simulink model "v09_twobit_mult"  (R2019b)
settings: Solver=FixedStepAuto  StartTime=0.0  StopTime=inf  FixedStep=1  MaxStep=1  RelTol=1e-3
libraries: simulink x4
settings Model: Creator=MARAT  LastModifiedBy=Marat
settings SFSimCC: CustomCodeUndefinedFunction=UseInterfaceOnly

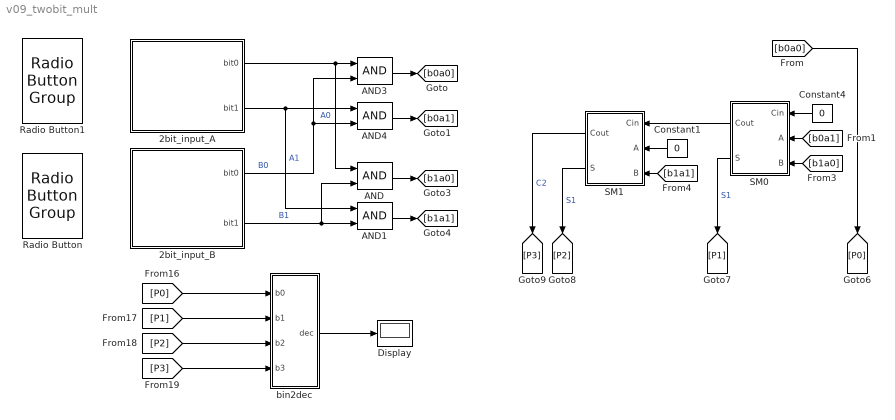
== system v09_twobit_mult ==
  2bit_input_A : Subsystem
      mask Display: image('images\sansA.png'); % Use "Edit Image" on toolstrip to change.
  2bit_input_B : Subsystem
      mask Display: image('images\sansB.png'); % Use "Edit Image" on toolstrip to change.
  AND{,1,3..4} (4 alike) : Logic  AllPortsSameDT=off  OutDataTypeStr=boolean
  Constant1 : Constant  Value=0  OutDataTypeStr=boolean
  Constant4 : Constant  Value=0  OutDataTypeStr=boolean
  Display : Display
  Radio Button : RadioButtonGroup  SelectedLabel=0
      settings: Values={{'0', '1', '2', '3'}, [0 1 2 3]}
  Radio Button1 : RadioButtonGroup  SelectedLabel=0
      settings: Values={{'0', '1', '2', '3'}, [0 1 2 3]}
  SM0 : Subsystem
  SM1 : Subsystem
  bin2dec : Subsystem
  wires:
  Constant4/1 -> SM0/1(Cin)
  [b0a0] -> [P0]
  2bit_input_A/1(bit0) -> AND/1, AND3/1  "A0"
  2bit_input_B/2(bit1) -> AND1/2, AND/2  "B1"
  [P0] -> bin2dec/1(b0)
  [P1] -> bin2dec/2(b1)
  [P2] -> bin2dec/3(b2)
  [P3] -> bin2dec/4(b3)
  bin2dec/1(dec) -> Display/1
  SM0/2(S) -> [P1]  "S1"
  2bit_input_A/2(bit1) -> AND1/1, AND4/1  "A1"
  2bit_input_B/1(bit0) -> AND3/2, AND4/2  "B0"
  AND3/1 -> [b0a0]
  AND4/1 -> [b0a1]
  AND1/1 -> [b1a1]
  AND/1 -> [b1a0]
  [b1a0] -> SM0/3(B)
  [b0a1] -> SM0/2(A)
  [b1a1] -> SM1/3(B)
  Constant1/1 -> SM1/2(A)
  SM0/1(Cout) -> SM1/1(Cin)
  SM1/2(S) -> [P2]  "S1"
  SM1/1(Cout) -> [P3]  "C2"

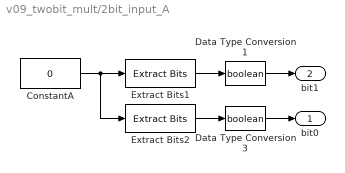
== system v09_twobit_mult/2bit_input_A ==
  ConstantA : Constant  Value=0  OutMin=0  OutMax=3  OutDataTypeStr=uint8
  Data Type Conversion1 : DataTypeConversion  OutDataTypeStr=boolean
  Data Type Conversion3 : DataTypeConversion  OutDataTypeStr=boolean
  Extract Bits1 : simulink/Logic and Bit Operations/Extract Bits  bitsToExtract=Range of bits  numBits=8  bitIdxRange=1  outScalingMode=Treat bit field as an integer
      settings: SourceProductName=Simulink
  Extract Bits2 : simulink/Logic and Bit Operations/Extract Bits  bitsToExtract=Range of bits  numBits=8  bitIdxRange=0  outScalingMode=Treat bit field as an integer
      settings: SourceProductName=Simulink
  bit0 : Outport
  bit1 : Outport  Port=2
  wires:
  ConstantA/1 -> Extract Bits2/1, Extract Bits1/1
  Extract Bits1/1 -> Data Type Conversion1/1
  Extract Bits2/1 -> Data Type Conversion3/1
  Data Type Conversion1/1 -> bit1/1
  Data Type Conversion3/1 -> bit0/1

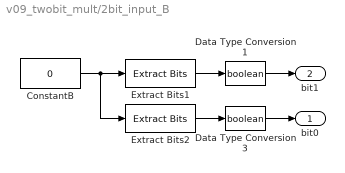
== system v09_twobit_mult/2bit_input_B ==
  ConstantB : Constant  Value=0  OutMin=0  OutMax=3  OutDataTypeStr=uint8
  Data Type Conversion1 : DataTypeConversion  OutDataTypeStr=boolean
  Data Type Conversion3 : DataTypeConversion  OutDataTypeStr=boolean
  Extract Bits1 : simulink/Logic and Bit Operations/Extract Bits  bitsToExtract=Range of bits  numBits=8  bitIdxRange=1  outScalingMode=Treat bit field as an integer
      settings: SourceProductName=Simulink
  Extract Bits2 : simulink/Logic and Bit Operations/Extract Bits  bitsToExtract=Range of bits  numBits=8  bitIdxRange=0  outScalingMode=Treat bit field as an integer
      settings: SourceProductName=Simulink
  bit0 : Outport
  bit1 : Outport  Port=2
  wires:
  Data Type Conversion3/1 -> bit0/1
  Data Type Conversion1/1 -> bit1/1
  Extract Bits2/1 -> Data Type Conversion3/1
  Extract Bits1/1 -> Data Type Conversion1/1
  ConstantB/1 -> Extract Bits1/1, Extract Bits2/1

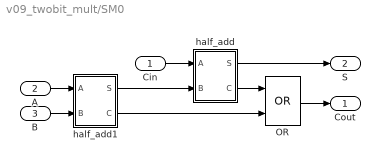
== system v09_twobit_mult/SM0 ==
  Cin : Inport
  A : Inport  Port=2
  B : Inport  Port=3
  OR : Logic  Operator=OR  AllPortsSameDT=off  OutDataTypeStr=boolean
  half_add : Subsystem
  half_add1 : Subsystem
  Cout : Outport
  S : Outport  Port=2
  wires:
  half_add/1(S) -> S/1
  A/1 -> half_add1/1(A)
  half_add/2(C) -> OR/1
  half_add1/1(S) -> half_add/2(B)
  B/1 -> half_add1/2(B)
  Cin/1 -> half_add/1(A)
  OR/1 -> Cout/1
  half_add1/2(C) -> OR/2

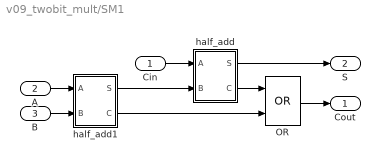
== system v09_twobit_mult/SM1 ==
  Cin : Inport
  A : Inport  Port=2
  B : Inport  Port=3
  OR : Logic  Operator=OR  AllPortsSameDT=off  OutDataTypeStr=boolean
  half_add : Subsystem
  half_add1 : Subsystem
  Cout : Outport
  S : Outport  Port=2
  wires:
  half_add1/2(C) -> OR/2
  OR/1 -> Cout/1
  Cin/1 -> half_add/1(A)
  B/1 -> half_add1/2(B)
  half_add1/1(S) -> half_add/2(B)
  half_add/2(C) -> OR/1
  A/1 -> half_add1/1(A)
  half_add/1(S) -> S/1

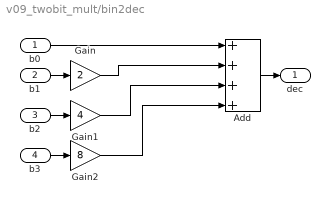
== system v09_twobit_mult/bin2dec ==
  b0 : Inport
  b1 : Inport  Port=2
  b2 : Inport  Port=3
  b3 : Inport  Port=4
  Add : Sum  Inputs=++++
  Gain : Gain  Gain=2
  Gain1 : Gain  Gain=4
  Gain2 : Gain  Gain=8
  dec : Outport
  wires:
  b1/1 -> Gain/1
  b3/1 -> Gain2/1
  b2/1 -> Gain1/1
  b0/1 -> Add/1
  Add/1 -> dec/1
  Gain/1 -> Add/2
  Gain1/1 -> Add/3
  Gain2/1 -> Add/4

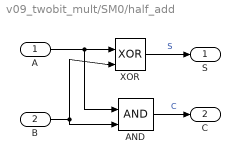
== system v09_twobit_mult/SM0/half_add ==
  A : Inport
  B : Inport  Port=2
  AND : Logic  IconShape=distinctive  AllPortsSameDT=off  OutDataTypeStr=boolean
  XOR : Logic  Operator=XOR  IconShape=distinctive  AllPortsSameDT=off  OutDataTypeStr=boolean
  S : Outport
  C : Outport  Port=2
  wires:
  XOR/1 -> S/1  "S"
  B/1 -> AND/2, XOR/2
  A/1 -> AND/1, XOR/1
  AND/1 -> C/1  "C"

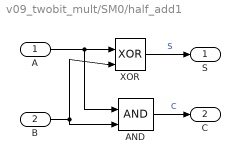
== system v09_twobit_mult/SM0/half_add1 ==
  A : Inport
  B : Inport  Port=2
  AND : Logic  IconShape=distinctive  AllPortsSameDT=off  OutDataTypeStr=boolean
  XOR : Logic  Operator=XOR  IconShape=distinctive  AllPortsSameDT=off  OutDataTypeStr=boolean
  S : Outport
  C : Outport  Port=2
  wires:
  AND/1 -> C/1  "C"
  A/1 -> XOR/1, AND/1
  B/1 -> XOR/2, AND/2
  XOR/1 -> S/1  "S"

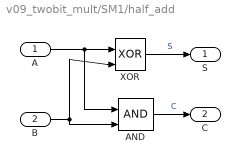
== system v09_twobit_mult/SM1/half_add ==
  A : Inport
  B : Inport  Port=2
  AND : Logic  IconShape=distinctive  AllPortsSameDT=off  OutDataTypeStr=boolean
  XOR : Logic  Operator=XOR  IconShape=distinctive  AllPortsSameDT=off  OutDataTypeStr=boolean
  S : Outport
  C : Outport  Port=2
  wires:
  AND/1 -> C/1  "C"
  A/1 -> XOR/1, AND/1
  B/1 -> XOR/2, AND/2
  XOR/1 -> S/1  "S"

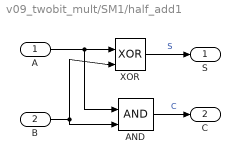
== system v09_twobit_mult/SM1/half_add1 ==
  A : Inport
  B : Inport  Port=2
  AND : Logic  IconShape=distinctive  AllPortsSameDT=off  OutDataTypeStr=boolean
  XOR : Logic  Operator=XOR  IconShape=distinctive  AllPortsSameDT=off  OutDataTypeStr=boolean
  S : Outport
  C : Outport  Port=2
  wires:
  XOR/1 -> S/1  "S"
  B/1 -> AND/2, XOR/2
  A/1 -> AND/1, XOR/1
  AND/1 -> C/1  "C"
